simulink model "q2sim"  (R2019b)
settings: Solver=VariableStepAuto  StartTime=0.0  StopTime=10.0  RelTol=1e-3
settings Model: Creator=samuelvenzi  LastModifiedBy=samuelvenzi

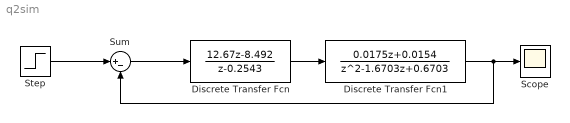
== system q2sim ==
  Discrete Transfer Fcn : DiscreteTransferFcn  Numerator=[12.67 -8.492]  Denominator=[1 -0.2543]  SampleTime=0.2
  Discrete Transfer Fcn1 : DiscreteTransferFcn  Numerator=[0.0175 0.0154]  Denominator=[1 -1.6703 +0.6703]  SampleTime=0.2
  Scope : Scope
  Step : Step  Time=0  SampleTime=0
  Sum : Sum  Inputs=|+-
  wires:
  Step/1 -> Sum/1
  Sum/1 -> Discrete Transfer Fcn/1
  Discrete Transfer Fcn/1 -> Discrete Transfer Fcn1/1
  Discrete Transfer Fcn1/1 -> Scope/1, Sum/2
